simulink model "lab11_sim"  (R2021a)
settings: Solver=VariableStepAuto  StartTime=0.0  StopTime=60  RelTol=1e-3
values from neighbouring files (symbols this model uses):
  A = [0 1 0 0 ... (first row only)    [lab11.m]
  Ac = J + H * F * M    [compensator_dinamic_stabilizator.m]
  B = [0; -1/(M*l); 0; 1/M]    [lab11.m]
  Bc = K + H * F * N    [compensator_dinamic_stabilizator.m]
  C = [1 0 0 0; 0 0 1 0]    [lab11.m]
  D = [0; 0]    [lab11.m]
undefined symbols (not defined in the file or in its folder): Fc, Gc
settings Model: Creator=Administrator  LastModifiedBy=Administrator

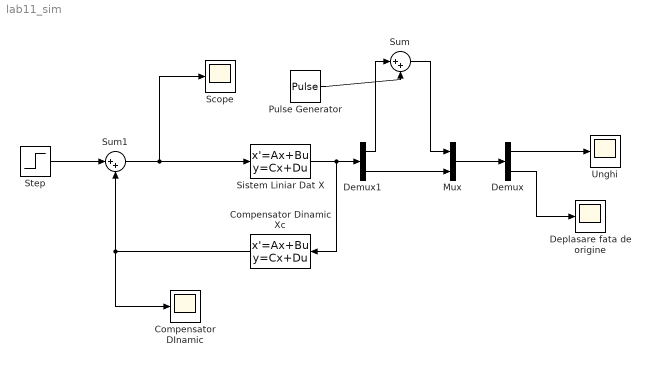
== system lab11_sim ==
  Compensator DInamic : Scope
  Compensator Dinamic Xc : StateSpace  A=Ac  B=Bc  C=Fc  D=Gc  InitialCondition=0
  Demux : Demux  Outputs=2
  Demux1 : Demux  Outputs=2
  Deplasare fata de origine : Scope
  Mux : Mux  Inputs=2
  Pulse Generator : DiscretePulseGenerator  PulseType=Time based  Amplitude=0.01  Period=10  PulseWidth=5
  Scope : Scope
  Sistem Liniar Dat X : StateSpace  A=A  B=B  C=C  D=D  InitialCondition=0
  Step : Step  Time=0  After=0.0001  SampleTime=0
  Sum : Sum  Inputs=|++
  Sum1 : Sum  Inputs=|++
  Unghi : Scope
  wires:
  Step/1 -> Sum1/1
  Sum1/1 -> Scope/1, Sistem Liniar Dat X/1
  Compensator Dinamic Xc/1 -> Compensator DInamic/1, Sum1/2
  Sistem Liniar Dat X/1 -> Demux1/1, Compensator Dinamic Xc/1
  Demux/1 -> Unghi/1
  Demux/2 -> Deplasare fata de origine/1
  Demux1/1 -> Sum/1
  Sum/1 -> Mux/1
  Mux/1 -> Demux/1
  Demux1/2 -> Mux/2
  Pulse Generator/1 -> Sum/2
